simulink model "two_wheeled"  (R2023a)
settings: Solver=VariableStepAuto  StartTime=0.0  StopTime=20  RelTol=1e-3
undefined symbols (not defined in the file): k_drag, m, magnitude, r
libraries: slpidlib x1
settings Model: Creator=jainam  LastModifiedBy=jainam

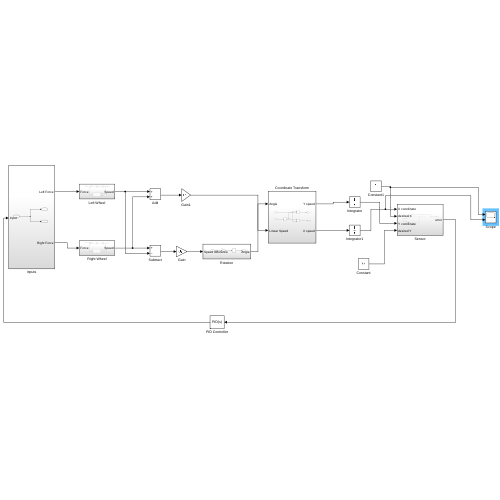
[thumbnail: Simulink's stored preview of the top-level diagram]
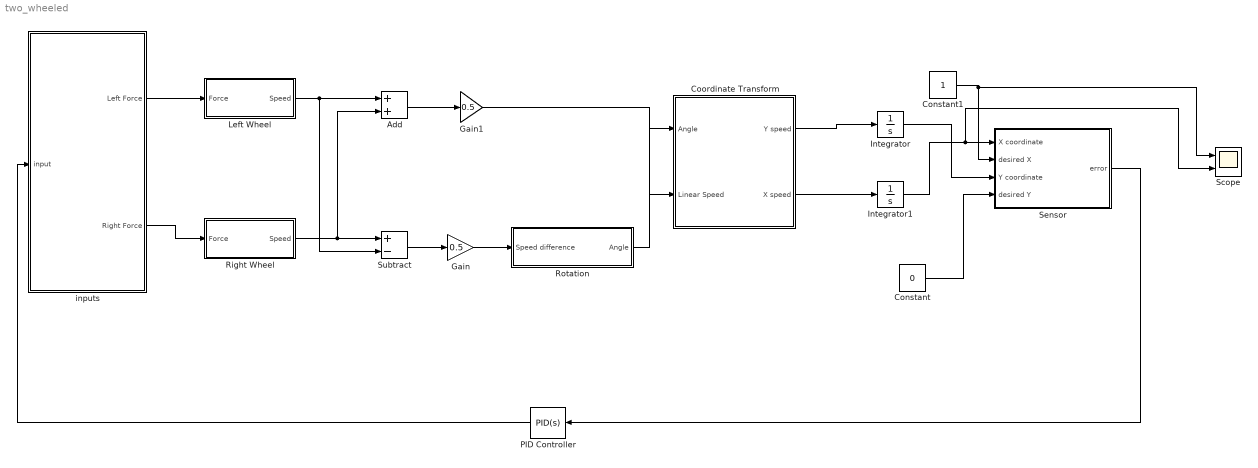
== system two_wheeled ==
  Add : Sum
  Constant : Constant  Value=0
  Constant1 : Constant
  Coordinate Transform : Subsystem
  Gain : Gain  Gain=0.5
  Gain1 : Gain  Gain=0.5
  Integrator : Integrator
  Integrator1 : Integrator
  Left Wheel : Subsystem
  PID Controller : slpidlib/PID Controller  Controller=PID  Form=Parallel  TimeDomain=Continuous-time  UseExternalTs=off  SampleTime=-1  IntegratorMethod=Forward Euler  FilterMethod=Forward Euler  ControllerParametersSource=internal  P=-29.0683086838108  I=-3.52642070962068  UseKiTs=off  D=-18.8666772667655  N=1733.8473494823  UseFilter=on  TunerSelectOption=Transfer Function Based (PID Tuner App)  InitialConditionSource=internal  InitialConditionForIntegrator=0  InitialConditionForFilter=0  DifferentiatorICPrevScaledInput=0  ExternalReset=none  TrackingMode=off  Kt=1  LimitOutput=off  SatLimitsSource=internal  UpperSaturationLimit=inf  LowerSaturationLimit=-inf  LinearizeAsGain=on  AntiWindupMode=none  Kb=1  LimitIntegrator=off  UpperIntegratorSaturationLimit=inf  LowerIntegratorSaturationLimit=-inf  POutMin=[]  POutMax=[]  IOutMin=[]  IOutMax=[]  DOutMin=[]  DOutMax=[]  NOutMin=[]  NOutMax=[]  SumOutMin=[]  SumOutMax=[]  SaturationOutMin=[]  SaturationOutMax=[]  PParamMin=[]  PParamMax=[]  IParamMin=[]  IParamMax=[]  DParamMin=[]  DParamMax=[]  NParamMin=[]  NParamMax=[]  KbParamMin=[]  KbParamMax=[]  KtParamMin=[]  KtParamMax=[]  KbOutMin=[]  KbOutMax=[]  KtOutMin=[]  KtOutMax=[]  IntegratorOutMin=[]  IntegratorOutMax=[]  FilterOutMin=[]  FilterOutMax=[]  SumI1OutMin=[]  SumI1OutMax=[]  SumI2OutMin=[]  SumI2OutMax=[]  SumI3OutMin=[]  SumI3OutMax=[]  SumI4OutMin=[]  SumI4OutMax=[]  SumDOutMin=[]  SumDOutMax=[]  DifferentiatorOutMin=[]  DifferentiatorOutMax=[]  FilterDiffOutCoefMin=[]  FilterDiffOutCoefMax=[]  ReciprocalOutMin=[]  ReciprocalOutMax=[]  SumDenOutMin=[]  SumDenOutMax=[]  SumNumOutMin=[]  SumNumOutMax=[]  DivideOutMin=[]  DivideOutMax=[]  UdiffTsProdOutMin=[]  UdiffTsProdOutMax=[]  NTsProdOutMin=[]  NTsProdOutMax=[]  UintegralTsProdOutMin=[]  UintegralTsProdOutMax=[]  UngainTsProdOutMin=[]  UngainTsProdOutMax=[]  ClampingZeroOutDataTypeStr=Inherit: Inherit via back propagation  ClampingZeroOutMin=[]  ClampingZeroOutMax=[]  FilterDenConstantOutDataTypeStr=Inherit: Inherit via back propagation  FilterDenConstantOutMin=[]  FilterDenConstantOutMax=[]  PCopyOutDataTypeStr=Inherit: Inherit via back propagation  PCopyOutMin=[]  PCopyOutMax=[]  NCopyOutDataTypeStr=Inherit: Inherit via back propagation  NCopyOutMin=[]  NCopyOutMax=[]  IntegratorContinuousStateAttributes=''  IntegratorStateMustResolveToSignalObject=off  IntegratorRTWStateStorageClass=Auto  FilterContinuousStateAttributes=''  FilterStateMustResolveToSignalObject=off  FilterRTWStateStorageClass=Auto  ParallelPVariant=InternalParameters  IdealPVariant=Disabled  IVariant=InternalParameters  DVariant=InternalParameters  IntegratorVariant=Continuous  SatVariant=Disabled  AWVariant=Passthrough  PCopyVariant=Disabled  TRVariant=Disabled  FdbkBlocksVariant=Forward  IdealPFdbkVariant=Disabled  SatFdbkVariant=Disabled  DerivativeFilterVariant=ContFilter  NVariant=InternalParameters  NCopyVariant=Disabled  FilterICVariant=InternalICsFilter  IntegratorICVariant=InternalICs  ExternalResetVariant=Disabled  TRSumVariant=Passthrough  SumFdbkVariant=Disabled  SumVariant=Sum_PID  TsampFilterVariant=InternalTs  TsampNgainVariant=Passthrough  TsampIntegralVariant=Disabled_SignalSpec  ExternalSaturationOutDataTypeStr=Inherit: Same as second input
  Right Wheel : Subsystem
  Rotation : Subsystem
  Scope : Scope  NumInputPorts=2
  Sensor : Subsystem
  Subtract : Sum  Inputs=+-
  inputs : Subsystem
  wires:
  Coordinate Transform/2(X speed) -> Integrator1/1
  Add/1 -> Gain1/1
  Gain1/1 -> Coordinate Transform/2(Linear Speed)
  Integrator/1 -> Sensor/3(Y coordinate)
  Gain/1 -> Rotation/1(Speed difference)
  Subtract/1 -> Gain/1
  inputs/1(Left Force) -> Left Wheel/1(Force)
  Rotation/1(Angle) -> Coordinate Transform/1(Angle)
  Left Wheel/1(Speed) -> Subtract/2, Add/1
  inputs/2(Right Force) -> Right Wheel/1(Force)
  Integrator1/1 -> Scope/2, Sensor/1(X coordinate)
  Right Wheel/1(Speed) -> Subtract/1, Add/2
  Coordinate Transform/1(Y speed) -> Integrator/1
  PID Controller/1 -> inputs/1(input)
  Sensor/1(error) -> PID Controller/1
  Constant1/1 -> Scope/1, Sensor/2(desired X)
  Constant/1 -> Sensor/4(desired Y)

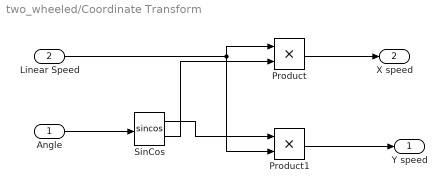
== system two_wheeled/Coordinate Transform ==
  Angle : Inport
  Linear Speed : Inport  Port=2
  Product : Product
  Product1 : Product
  SinCos : Trigonometry  Operator=sincos
  Y speed : Outport
  X speed : Outport  Port=2
  wires:
  Angle/1 -> SinCos/1
  Product1/1 -> Y speed/1
  Linear Speed/1 -> Product1/2, Product/1
  Product/1 -> X speed/1
  SinCos/1 -> Product1/1
  SinCos/2 -> Product/2

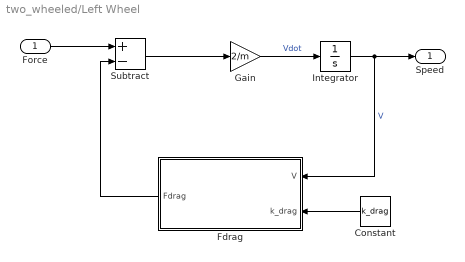
== system two_wheeled/Left Wheel ==
  Force : Inport
  " Fdrag" : MATLAB Function  TreatAsAtomicUnit=on
  Constant : Constant  Value=k_drag
  Gain : Gain  Gain=2/m
  Integrator : Integrator
  Subtract : Sum  Inputs=+-
  Speed : Outport
  wires:
  Force/1 -> Subtract/1
  Subtract/1 -> Gain/1
  Gain/1 -> Integrator/1  "Vdot"
  Integrator/1 -> " Fdrag"/1(V), Speed/1  "V"
  " Fdrag"/1(Fdrag) -> Subtract/2
  Constant/1 -> " Fdrag"/2(k_drag)

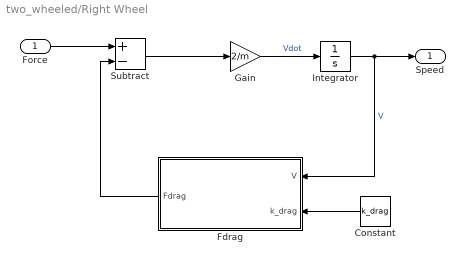
== system two_wheeled/Right Wheel ==
  Force : Inport
  " Fdrag" : MATLAB Function  TreatAsAtomicUnit=on
  Constant : Constant  Value=k_drag
  Gain : Gain  Gain=2/m
  Integrator : Integrator
  Subtract : Sum  Inputs=+-
  Speed : Outport
  wires:
  Force/1 -> Subtract/1
  Subtract/1 -> Gain/1
  Gain/1 -> Integrator/1  "Vdot"
  Integrator/1 -> " Fdrag"/1(V), Speed/1  "V"
  " Fdrag"/1(Fdrag) -> Subtract/2
  Constant/1 -> " Fdrag"/2(k_drag)

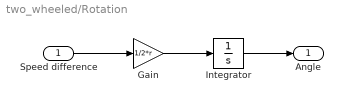
== system two_wheeled/Rotation ==
  Speed difference : Inport
  Gain : Gain  Gain=1/2*r
  Integrator : Integrator
  Angle : Outport
  wires:
  Speed difference/1 -> Gain/1
  Gain/1 -> Integrator/1
  Integrator/1 -> Angle/1

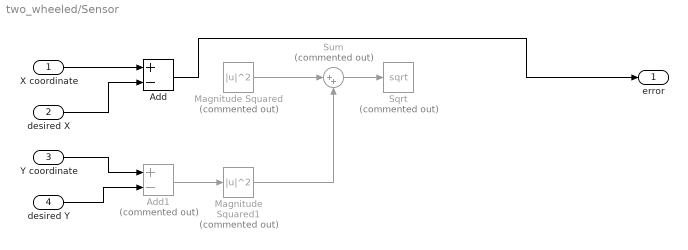
== system two_wheeled/Sensor ==
  X coordinate : Inport
  desired X : Inport  Port=2
  Y coordinate : Inport  Port=3
  desired Y : Inport  Port=4
  Add : Sum  Inputs=+-
  Add1 : Sum  Commented=on  Inputs=+-
  Magnitude Squared : Math  Commented=on  Operator=magnitude^2
  Magnitude Squared1 : Math  Commented=on  Operator=magnitude^2
  Sqrt : Sqrt  Commented=on
  Sum : Sum  Commented=on  Inputs=|++
  error : Outport
  wires:
  Y coordinate/1 -> Add1/1
  desired Y/1 -> Add1/2
  X coordinate/1 -> Add/1
  desired X/1 -> Add/2
  Add1/1 -> Magnitude Squared1/1
  Magnitude Squared/1 -> Sum/1
  Magnitude Squared1/1 -> Sum/2
  Sum/1 -> Sqrt/1
  Add/1 -> error/1

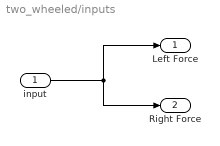
== system two_wheeled/inputs ==
  input : Inport
  Left Force : Outport
  Right Force : Outport  Port=2
  wires:
  input/1 -> Left Force/1, Right Force/1

== matlab function two_wheeled/Right Wheel/ Fdrag ==
  data: V input; Fdrag output; k_drag input
function Fdrag = get_fdrag(V,k_drag)

Fdrag = k_drag*V*abs(V);

== matlab function two_wheeled/Left Wheel/ Fdrag ==
  data: V input; Fdrag output; k_drag input
function Fdrag = get_fdrag(V,k_drag)

Fdrag = k_drag*V*abs(V);
